simulink model "smith_water_cr"  (R2021a)
settings: Solver=VariableStepAuto  StartTime=0.0  StopTime=610  RelTol=1e-3
undefined symbols (not defined in the file): params
libraries: cstblocks x6, simulink x1
settings Model: Creator=victo  LastModifiedBy=victo

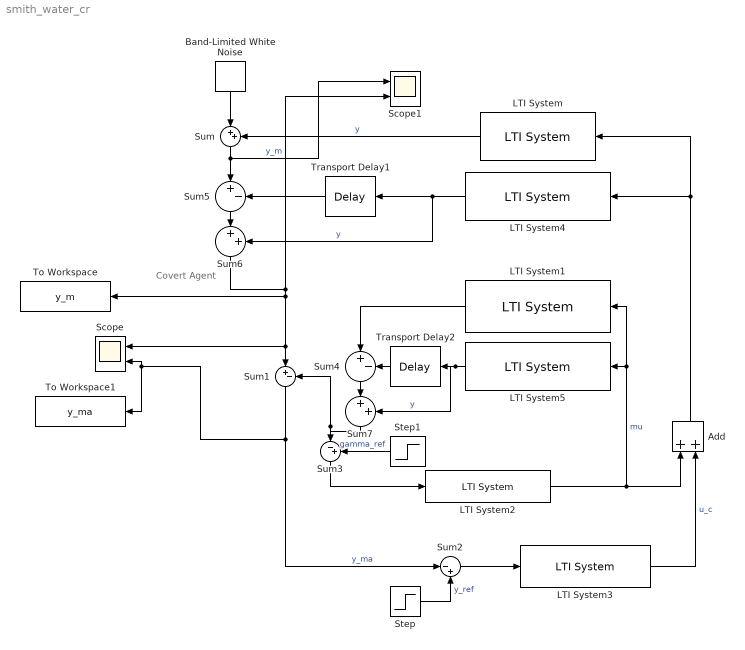
== system smith_water_cr ==
  note: Covert Agent
  Add : Sum
  Band-Limited White Noise : simulink/Sources/Band-Limited White Noise  Cov=params.noise_power  Ts=params.Ts  seed=params.seed
  LTI System : cstblocks/LTI System  sys=params.nominal_plant  IC=[]
  LTI System1 : cstblocks/LTI System  sys=params.plant_model_attacker  IC=[]
  LTI System2 : cstblocks/LTI System  sys=params.covert_controller  IC=[]
  LTI System3 : cstblocks/LTI System  sys=params.nominal_controller  IC=[]
  LTI System4 : cstblocks/LTI System  sys=params.plant_model_no_delay  IC=[]
  LTI System5 : cstblocks/LTI System  sys=params.plant_model_no_delay_attacker  IC=[]
  Scope : Scope  NumInputPorts=2
  Scope1 : Scope  NumInputPorts=2
  Step : Step  Time=params.y_ref_start  After=params.y_ref_value  SampleTime=0
  Step1 : Step  Time=params.gamma_ref_start  After=params.gamma_ref_value  SampleTime=0
  Sum : Sum  Inputs=|++
  Sum1 : Sum  Inputs=|+-
  Sum2 : Sum  Inputs=|-+
  Sum3 : Sum  Inputs=|-+
  Sum4 : Sum  Inputs=|+-
  Sum5 : Sum  Inputs=|+-
  Sum6 : Sum  Inputs=|++
  Sum7 : Sum  Inputs=|++
  To Workspace : ToWorkspace  VariableName=y_m  SaveFormat=Timeseries  SampleTime=params.Ts
  To Workspace1 : ToWorkspace  VariableName=y_ma  SaveFormat=Timeseries  SampleTime=params.Ts
  Transport Delay1 : TransportDelay  DelayTime=0.29  BufferSize=8192
  Transport Delay2 : TransportDelay  DelayTime=0.29  BufferSize=8192
  wires:
  Step/1 -> Sum2/2  "y_ref"
  Sum3/1 -> LTI System2/1
  Sum2/1 -> LTI System3/1
  LTI System3/1 -> Add/2  "u_c"
  Sum1/1 -> To Workspace1/1, Scope/2, Sum2/1  "y_ma"
  LTI System2/1 -> LTI System5/1, LTI System1/1, Add/1  "mu"
  Step1/1 -> Sum3/2  "gamma_ref"
  Band-Limited White Noise/1 -> Sum/1
  Add/1 -> LTI System4/1, LTI System/1
  LTI System4/1 -> Sum6/2, Transport Delay1/1  "y"
  Transport Delay1/1 -> Sum5/2
  Sum5/1 -> Sum6/1
  LTI System5/1 -> Sum7/2, Transport Delay2/1  "y"
  Transport Delay2/1 -> Sum4/2
  LTI System1/1 -> Sum4/1
  Sum4/1 -> Sum7/1
  Sum7/1 -> Sum1/2, Sum3/1
  Sum/1 -> Scope1/1, Sum5/1  "y_m"
  LTI System/1 -> Sum/2  "y"
  Sum6/1 -> Sum1/1, Scope/1, To Workspace/1, Scope1/2
